simulink model "Day6_lab"  (R2021a)
settings: Solver=VariableStepAuto  StartTime=0.0  StopTime=10.0  RelTol=1e-3
values from neighbouring files (symbols this model uses):
  a1 = input('enter acc1: ')    [Day10.m]
  a2 = input('enter acc2: ')    [Day10.m]
undefined symbols (not defined in the file or in its folder): a3
settings Model: Creator=Kanha  LastModifiedBy=Kanha

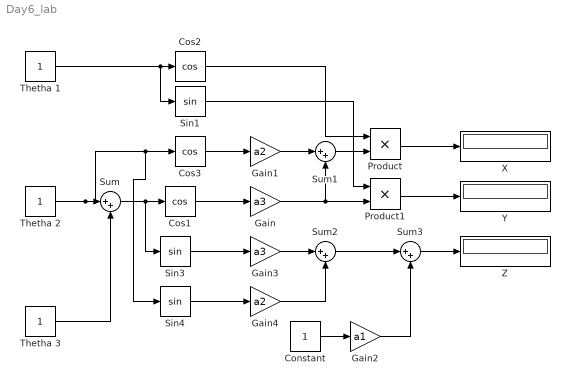
== system Day6_lab ==
  Constant : Constant
  Cos1 : Trigonometry  Operator=cos
  Cos2 : Trigonometry  Operator=cos
  Cos3 : Trigonometry  Operator=cos
  Gain : Gain  Gain=a3
  Gain1 : Gain  Gain=a2
  Gain2 : Gain  Gain=a1
  Gain3 : Gain  Gain=a3
  Gain4 : Gain  Gain=a2
  Product : Product
  Product1 : Product
  Sin1 : Trigonometry
  Sin3 : Trigonometry
  Sin4 : Trigonometry
  Sum{,1..3} (4 alike) : Sum  Inputs=|++
  Thetha 1 : Constant
  Thetha 2 : Constant
  Thetha 3 : Constant
  X : Display
  Y : Display
  Z : Display
  wires:
  Thetha 2/1 -> Cos3/1, Sin4/1, Sum/1
  Thetha 3/1 -> Sum/2
  Sum/1 -> Sin3/1, Cos1/1
  Cos1/1 -> Gain/1
  Gain1/1 -> Sum1/1
  Gain/1 -> Product1/2, Sum1/2
  Cos3/1 -> Gain1/1
  Sum1/1 -> Product/2
  Thetha 1/1 -> Sin1/1, Cos2/1
  Cos2/1 -> Product/1
  Product/1 -> X/1
  Sin1/1 -> Product1/1
  Product1/1 -> Y/1
  Sin3/1 -> Gain3/1
  Sin4/1 -> Gain4/1
  Gain3/1 -> Sum2/1
  Gain4/1 -> Sum2/2
  Constant/1 -> Gain2/1
  Gain2/1 -> Sum3/2
  Sum2/1 -> Sum3/1
  Sum3/1 -> Z/1
